simulink model "Glenn_final_modified_v1"  (R2019b)
settings: Solver=FixedStepDiscrete  StartTime=0.0  StopTime=Inf  FixedStep=0.01  RelTol=1e-3  EnableMultiTasking=on
values from neighbouring files (symbols this model uses):
  myParam = Simulink.Parameter    [activeCollisionCheck_truckRun.m]    (also in joystick.m)
  myParam1 = Simulink.Parameter    [activeCollisionCheck_truckRun.m]    (also in joystick.m)
  myParam2 = Simulink.Parameter    [activeCollisionCheck_truckRun.m]    (also in joystick.m)
undefined symbols (not defined in the file or in its folder): Angular, Linear
libraries: robotlib x3, simulink x1
settings Model: SimulationMode=external  Creator=The MathWorks, Inc.  LastModifiedBy=gdubbelman
settings DataIOCC: SaveFinalState=on  SaveFormat=Array  SaveState=on  SignalLoggingName=poses  LoggingFileName=pose.mat
settings OptimizationCC: ZeroExternalMemoryAtStartup=off  ZeroInternalMemoryAtStartup=off  LifeSpan=Inf  MaxStackSize=64
settings DebuggingCC: SolverPrmCheckMsg=warning  SFUnexpectedBacktrackingDiag=warning  SFNoUnconditionalDefaultTransitionDiag=warning  SFExecutionAtInitializationDiag=none  ArithmeticOperatorsInVariantConditions=warning
settings HardwareCC: ProdBitPerPointer=32  ProdBitPerSizeT=32  ProdBitPerPtrDiffT=32  ProdLargestAtomicFloat=None  ProdIntDivRoundTo=Undefined  ProdEndianess=Unspecified  ProdWordSize=32  ProdHWDeviceType=Generic->Unspecified (assume 32-bit Generic)  UseEmbeddedCoderFeatures=off
settings ModelReferenceCC: UpdateModelReferenceTargets=Force  PropagateSignalLabelsOutOfModel=off
settings SFSimCC: SimUseLocalCustomCode=off  CustomCodeUndefinedFunction=UseInterfaceOnly
settings RTWCC: SystemTargetFile=ert.tlc  HardwareBoard=Robot Operating System (ROS)  TLCOptions=-aInlineSetEventsForThisBaseRateFcn=TLC_FALSE -aSuppressMultiTaskScheduler=TLC_FALSE -aRateBasedStepFcn=0  TemplateMakefile=ert_default_tmf  RTWUseLocalCustomCode=off  Toolchain=Catkin  TargetLang=C++
settings CodeAppCC: StateflowObjectComments=on
settings ERTTargetCC: MultiwordLength=2048  ERTCustomFileBanners=off  SupportContinuousTime=on  SupportNonInlinedSFcns=on  RemoveResetFunc=off  SupportVariableSizeSignals=on  ModelStepFunctionPrototypeControlCompliant=off  ExtMode=on  ExtModeMexArgs='192.168.0.200' 0 17725  ERTSrcFileBannerTemplate=codertarget_code_template.cgt  ERTHdrFileBannerTemplate=codertarget_code_template.cgt  ERTDataSrcFileTemplate=codertarget_code_template.cgt  ERTDataHdrFileTemplate=codertarget_code_template.cgt  ConvertIfToSwitch=off  SuppressUnreachableDefaultCases=off
settings ConfigComp: CovMetricSettings=dw  CovHtmlReporting=on  CovSaveCumulativeToWorkspaceVar=on  CovSaveSingleToWorkspaceVar=on  CovExternalEMLEnable=off  CovSFcnEnable=off

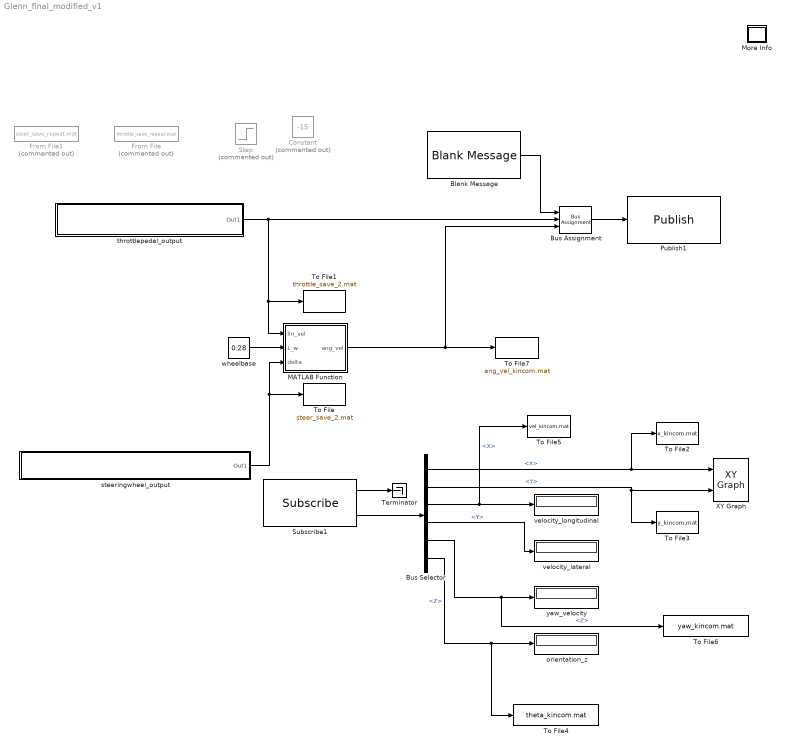
== system Glenn_final_modified_v1 ==
  Blank Message : robotlib/Blank Message  messageClass=Message  entityType=geometry_msgs/Twist  messageType=geometry_msgs/Twist  SampleTime=-1
      settings: SourceProductName=ROS Toolbox
  Bus Assignment : BusAssignment  DialogController=Simulink.DDGSource_BusAssignment  AssignedSignals=Linear.X,Angular.Z
  Bus Selector : BusSelector  DialogController=Simulink.DDGSource_BusSelector  OutputSignals=Pose.Pose.Position.X,Pose.Pose.Position.Y,Twist.Twist.Linear.X,Twist.Twist.Linear.Y,Twist.Twist.Angular.Z,Pose.Pose.Orientation.Z
  Constant : Constant  Commented=on  Value=-15
  From File : FromFile  Commented=on  FileName=throttle_save_repeat.mat
  From File1 : FromFile  Commented=on  FileName=steer_save_repeat.mat
  MATLAB Function : MATLAB Function  TreatAsAtomicUnit=on
  More Info : Subsystem
      settings: OpenFcn=showdemo(bdroot(gcb))
      mask Display: disp('?')
  Publish1 : robotlib/Publish  topicSource=Select from ROS network  topic=/cmd_vel  messageType=geometry_msgs/Twist  messageQueueLength=105
      settings: SourceProductName=ROS Toolbox
  Step : Step  Commented=on  Time=10  After=0.5  SampleTime=0
  Subscribe1 : robotlib/Subscribe  topicSource=Select from ROS network  topic=/odom  messageType=nav_msgs/Odometry  sampleTime=-1  messageQueueLength=51
      settings: SourceProductName=ROS Toolbox
  Terminator : Terminator
  To File : ToFile  Filename=steer_save_2.mat  MatrixName=steer_save
  To File1 : ToFile  Filename=throttle_save_2.mat  MatrixName=throttle_save
  To File2 : ToFile  Filename=x_kincom.mat  MatrixName=x_line
  To File3 : ToFile  Filename=y_kincom.mat  MatrixName=y_line
  To File4 : ToFile  Filename=theta_kincom.mat  MatrixName=theta
  To File5 : ToFile  Filename=vel_kincom.mat  MatrixName=vel
  To File6 : ToFile  Filename=yaw_kincom.mat  MatrixName=yaw
  To File7 : ToFile  Filename=ang_vel_kincom.mat  MatrixName=ang_vel
  XY Graph : simulink/Sinks/XY Graph  xmin=-10  xmax=10  ymin=-10  ymax=10  st=-1
  orientation_z : Display
  steeringwheel_output : Subsystem
  throttlepedal_output : Subsystem
  velocity_lateral : Display
  velocity_longitudinal : Display
  wheelbase : Constant  Value=0.28
  yaw_velocity : Display
  wires:
  Bus Assignment/1 -> Publish1/1
  Blank Message/1 -> Bus Assignment/1
  Bus Selector/2 -> To File3/1, XY Graph/2  "<Y>"
  MATLAB Function/1(ang_vel) -> Bus Assignment/3, To File7/1
  Subscribe1/1 -> Terminator/1
  wheelbase/1 -> MATLAB Function/2(L_w)
  steeringwheel_output/1(Out1) -> To File/1, MATLAB Function/3(delta)
  throttlepedal_output/1(Out1) -> Bus Assignment/2, MATLAB Function/1(lin_vel), To File1/1
  Subscribe1/2 -> Bus Selector/1
  Bus Selector/1 -> XY Graph/1, To File2/1  "<X>"
  Bus Selector/3 -> To File5/1, velocity_longitudinal/1  "<X>"
  Bus Selector/4 -> velocity_lateral/1  "<Y>"
  Bus Selector/6 -> To File4/1, orientation_z/1  "<Z>"
  Bus Selector/5 -> To File6/1, yaw_velocity/1  "<Z>"

== system Glenn_final_modified_v1/More Info ==

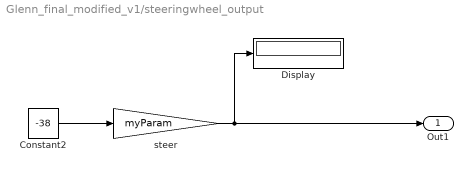
== system Glenn_final_modified_v1/steeringwheel_output ==
  Constant2 : Constant  Value=-38
  Display : Display
  "steer " : Gain  Gain=myParam
  Out1 : Outport
  wires:
  Constant2/1 -> "steer "/1
  "steer "/1 -> Out1/1, Display/1

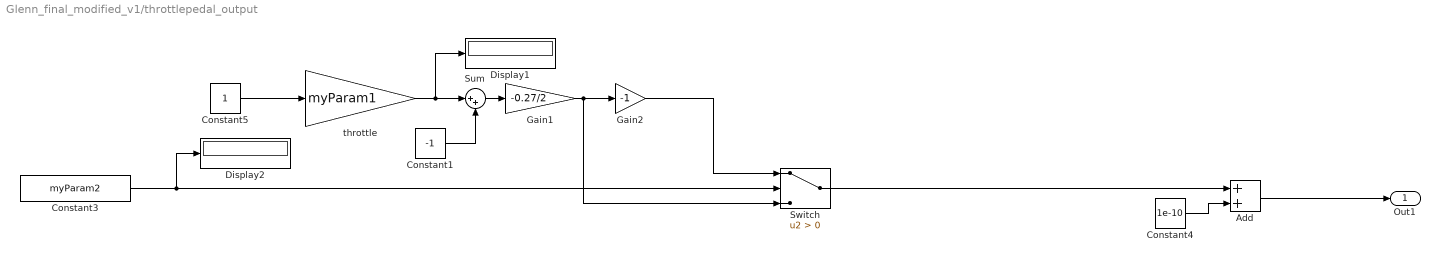
== system Glenn_final_modified_v1/throttlepedal_output ==
  Add : Sum
  Constant1 : Constant  Value=-1
  Constant3 : Constant  Value=myParam2
  Constant4 : Constant  Value=1e-10
  Constant5 : Constant
  Display1 : Display
  Display2 : Display
  Gain1 : Gain  Gain=-0.27/2
  Gain2 : Gain  Gain=-1
  Sum : Sum  Inputs=|++
  Switch : Switch  Criteria=u2 > Threshold
  throttle : Gain  Gain=myParam1
  Out1 : Outport
  wires:
  Sum/1 -> Gain1/1
  throttle/1 -> Display1/1, Sum/1
  Constant3/1 -> Display2/1, Switch/2
  Constant1/1 -> Sum/2
  Constant5/1 -> throttle/1
  Gain1/1 -> Gain2/1, Switch/3
  Constant4/1 -> Add/2
  Add/1 -> Out1/1
  Gain2/1 -> Switch/1
  Switch/1 -> Add/1

== matlab function Glenn_final_modified_v1/MATLAB Function ==
  data: lin_vel input; ang_vel output; L_w input; delta input
function ang_vel = fcn(lin_vel,L_w,delta)

ang_vel=lin_vel/(L_w/tand(delta));
